simulink library "vmc"  (R2021b)
settings: Solver=VariableStepAuto  StartTime=0.0  StopTime=10.0  RelTol=1e-3
undefined symbols (not defined in the file): AVMC_ACCDeltaTqGradeGn_X_deg, AVMC_ACCDeltaTqIGain4OVRD_X_kph, AVMC_ACCDeltaTqIGain4OVRD_Y_mps2, AVMC_ACCDeltaTqIGain_X_kph, AVMC_ACCDeltaTqIGain_Y_mps2, AVMC_ACCDeltaTqPGain_X_kph, AVMC_ACCDeltaTqPGain_Y_kph, AVMC_ACCGradeofst_X_G, AVMC_ACCGradeofst_Y_pct, AVMC_ACCLoSpdTqLoLim4JP_X_kph, AVMC_ACCLoSpdTqLoLim4JP_Y_deg, AVMC_ACCLoSpdTqLowerLim_X_kph, AVMC_ACCLoSpdTqLowerLim_Y_deg, AVMC_ACCReqAccelGain_X_mps2, AVMC_ACCReqAccelGain_Y_enum, AVMC_ADSPosGFBDeltaTq_X_kph, AVMC_ADSPosGFBDeltaTq_Y_mps2, AVMC_AggressJerkPCT4AT_X_kph, AVMC_AggressJerkPCT_X_kph, AVMC_AggressLimitPCT4AT_X_kph, AVMC_AggressLimitPCT_X_kph, AVMC_DECGradeofst_X_G, AVMC_DECGradeofst_Y_pct, AVMC_DISCDeltaTqIGain_X_kph, AVMC_DISCDeltaTqIGain_Y_mps2, AVMC_DISCDeltaTqPGain_X_kph, AVMC_DISCDeltaTqPGain_Y_kph, AVMC_EPSForceSelect_X_enum, AVMC_EPSForceSelect_Y_enum, AVMC_EPSForceSelectD21_X_enum, AVMC_EPSForceSelectD21_Y_enum, AVMC_ESCRegenOut_X_kph, AVMC_ESCRegenOut_Y_Deg, AVMC_ESCRegenOutEnSpd_X_Deg, AVMC_EstPitchSlopeTs_X_kph, AVMC_GradeCompFlt_X_kph, AVMC_GyroYBandLo_X_Gps, AVMC_HoldResTq_X_kph, AVMC_ISOAccLimit_X_mps, AVMC_ISODecLimit_X_mps, AVMC_ISOJerk_X_mps, AVMC_LatESCRegenOut_X_kph, AVMC_LatESCRegenOut_Y_Deg, AVMC_LongAccDeadZone_X_kph, AVMC_LongAccFiltTsforP2_X_Gps, AVMC_MCPresBaseTq_X_bar, AVMC_MSAPedalOvrd_X_kph, AVMC_MSASpdBand_X_kph, AVMC_MSATqDownEndTq_X_kph, AVMC_MSATqDownTime_X_kph, AVMC_NegZCHoldTq_X_kph, AVMC_OPDDisSlideRate_X_Deg, AVMC_OVRD2ActSR2FCMCMD_X_mps2, AVMC_PedalTqRWhlRatio_X_Nm, AVMC_PedalTqRWhlRatio_Y_gps, AVMC_PedalTqRWhlSlipGain_X_rat, AVMC_PedalTqRWhlSlipGain_Y_kph, AVMC_PedalTqRWhSTRGGain_X_deg, AVMC_PedalTqRWhSTRGGain_Y_kph, AVMC_PosZCHoldTq_X_kph ... (+593)
libraries: hcu_lib x143, simulink x96, tqr x4, $bdroot x1, simulink_extras x1
(part 14 of 17)

== system vmc/VMC/VMC/Slide Rate  Calculation/Coordination ==
  VTQD_AfterAvailableTqDemFr_Nm : Inport
  VTQD_EquivAccPedalSWSta_flg : Inport  Port=2
  VINP_BrkPedalPos_pct : Inport  Port=3
  VVMC_PredictVehSpd_kph : Inport  Port=4
  VVMC_VehicleSpeed_kph : Inport  Port=5
  task_time_s : Inport  Port=6
  VINP_BrkSwSta_flg : Inport  Port=7
  VVMC_RawWhlSpdSlideRate_pct : Inport  Port=8
  VVMC_LFWhlSpdSlideRate_pct : Inport  Port=9
  VVMC_RFWhlSpdSlideRate_pct : Inport  Port=10
  VVMC_LRWhlSpdSlideRate_pct : Inport  Port=11
  VVMC_RRWhlSpdSlideRate_pct : Inport  Port=12
  VVMC_4WhlSpdSlideRate_pct : Inport  Port=13
  VVMC_LF4WhlSpdSlideRate_pct : Inport  Port=14
  VVMC_RF4WhlSpdSlideRate_pct : Inport  Port=15
  VVMC_LR4WhlSpdSlideRate_pct : Inport  Port=16
  VVMC_RR4WhlSpdSlideRate_pct : Inport  Port=17
  VVMC_AllWhlSkid_flg : Inport  Port=18
  VTQD_AfterAvailableTqDemRr_Nm : Inport  Port=19
  VVMC_AltWhlSlideRate_pct : Inport  Port=20
  VTQD_VehActSpd_kph : Inport  Port=21
  VTQD_RegenMode_enum : Inport  Port=22
  VVMC_EstSlope_Deg : Inport  Port=23
  AND : Logic  Inputs=4  AllPortsSameDT=off  OutDataTypeStr=boolean
  AND1 : Logic  AllPortsSameDT=off  OutDataTypeStr=boolean
  AND2 : Logic  AllPortsSameDT=off  OutDataTypeStr=boolean
  AND3 : Logic  Inputs=5  AllPortsSameDT=off  OutDataTypeStr=boolean
  Abs : Abs
  Abs1 : Abs
  Add : Sum  Inputs=+-
  Constant1 : Constant  Value=KVMC_WhlSlideEnDetTq_Nm
  Constant10 : Constant  Value=KVMC_WhlSlideEnDetTq_Nm
  Constant11 : Constant  Value=KVMC_AltWheelSlideRateSW_flg
  Constant{12..16} (5 alike) : Constant  Value=KVMC_CalWhleelSlideTs_c
  Constant17 : Constant  Value=KVMC_AltWheelSlideRateSW_flg
  Constant18 : Constant  Value=ZERO_FLOAT
  Constant19 : Constant  Value=KVMC_OPDDisSlideRateSpd_kph
  Constant2 : Constant  Value=KVMC_WhlSlideEnDetBrkPedal_pct
  Constant20 : Constant  Value=ENUM_REGENLEVEL_OPD
  Constant21 : Constant  Value=ZERO_FLOAT
  Constant{6..9,22} (5 alike) : Constant  Value=ONE_FLOAT
  Constant3 : Constant  Value=KVMC_4WhlSlideVehSpdDev_kph
  Constant4 : Constant  Value=KVMC_WhlSlideEnDetVehSpd_kph
  Constant5 : Constant  Value=KVMC_4WhleelSlideDetTime_s
  DelayEnable : hcu_lib/Basic_Blocks/DelayEnable
  Equal : RelationalOperator  Operator===  OutDataTypeStr=boolean  RndMeth=Simplest
  FirstOrderFilter{,1..4} (5 alike) : hcu_lib/Basic_Blocks/FirstOrderFilter
  MVMC_OPDDisSlideRate_Y_pct : Lookup_n-D  NumberOfTableDimensions=1  BreakpointsForDimension1=AVMC_OPDDisSlideRate_X_Deg  Table=MVMC_OPDDisSlideRate_Y_pct  InternalRulePriority=Speed  RndMeth=Simplest  InputSameDT=on
  NOT{,1..3} (4 alike) : Logic  Operator=NOT  AllPortsSameDT=off  OutDataTypeStr=boolean
  OR : Logic  Operator=OR  Inputs=3  AllPortsSameDT=off  OutDataTypeStr=boolean
  Relational Operator{,1,3..4,7} (5 alike) : RelationalOperator  OutDataTypeStr=boolean  RndMeth=Simplest
  Relational Operator2 : RelationalOperator  Operator=<  OutDataTypeStr=boolean  RndMeth=Simplest
  Relational Operator5 : RelationalOperator  Operator=<=  OutDataTypeStr=boolean  RndMeth=Simplest
  Relational Operator6 : RelationalOperator  Operator=<  OutDataTypeStr=boolean  RndMeth=Simplest
  Relay : Relay  OnSwitchValue=KTQD_OPDHoldGradeUp_Deg  OffSwitchValue=KTQD_OPDHoldGradeDown_Deg  OutDataTypeStr=boolean
  Switch{,1..11} (12 alike) : Switch  Criteria=u2 > Threshold
  VVMC_ActMaxSlideRate_pct : Outport
  VVMC_ActLFSlideRate_pct : Outport  Port=2
  VVMC_ActRFSlideRate_pct : Outport  Port=3
  VVMC_ActLRSlideRate_pct : Outport  Port=4
  VVMC_ActRRSlideRate_pct : Outport  Port=5
  wires:
  [VVMC_SlideRateEnCal_flg] -> Switch9/2
  [VVMC_SlideRateEnCal_flg] -> Switch7/2
  [VVMC_SlideRateEnCal_flg] -> Switch5/2
  [VVMC_SlideRateEnCal_flg] -> Switch3/2
  [VVMC_SlideRateEnCal_flg] -> Switch1/2
  [VVMC_EstSlope_Deg] -> Relay/1
  Relay/1 -> NOT3/1
  NOT3/1 -> AND3/5
  Relational Operator7/1 -> AND3/4
  [VTQD_VehActSpd_kph] -> Relational Operator7/1
  Constant22/1 -> Relational Operator7/2
  Constant21/1 -> Switch11/1
  [VVMC_OPDDisSlideRate_flg] -> Switch11/2
  Switch11/1 -> [VVMC_ActMaxSlideRate_pct]  "VVMC_ActMaxSlideRate_pct"
  FirstOrderFilter/1 -> Switch11/3, [VVMC_IntMaxSlideRate_pct]  "VVMC_IntMaxSlideRate_pct"
  Abs1/1 -> Relational Operator6/1
  [VVMC_IntMaxSlideRate_pct] -> Abs1/1
  AND3/1 -> [VVMC_OPDDisSlideRate_flg]  "VVMC_OPDDisSlideRate_flg"
  Relational Operator6/1 -> AND3/3
  Equal/1 -> AND3/2
  Relational Operator5/1 -> AND3/1
  MVMC_OPDDisSlideRate_Y_pct/1 -> Relational Operator6/2  "VVMC_OPDDisSlideRate_pct"
  [VVMC_EstSlope_Deg] -> MVMC_OPDDisSlideRate_Y_pct/1
  Constant20/1 -> Equal/2
  [VTQD_RegenMode_enum] -> Equal/1
  Constant19/1 -> Relational Operator5/2
  [VTQD_VehActSpd_kph] -> Relational Operator5/1
  VTQD_VehActSpd_kph/1 -> [VTQD_VehActSpd_kph]
  VTQD_RegenMode_enum/1 -> [VTQD_RegenMode_enum]
  VVMC_EstSlope_Deg/1 -> [VVMC_EstSlope_Deg]
  AND2/1 -> Switch/2
  NOT2/1 -> AND2/2
  Constant17/1 -> NOT2/1
  [task_time_s] -> FirstOrderFilter4/2
  Constant16/1 -> FirstOrderFilter4/3
  [task_time_s] -> FirstOrderFilter3/2
  Constant15/1 -> FirstOrderFilter3/3
  Constant14/1 -> FirstOrderFilter2/3
  [task_time_s] -> FirstOrderFilter2/2
  Constant13/1 -> FirstOrderFilter1/3
  [task_time_s] -> FirstOrderFilter1/2
  [task_time_s] -> FirstOrderFilter/2
  Constant12/1 -> FirstOrderFilter/3
  FirstOrderFilter4/1 -> [VVMC_ActRRSlideRate_pct]  "VVMC_ActRRSlideRate_pct"
  Switch9/1 -> FirstOrderFilter4/1
  FirstOrderFilter3/1 -> [VVMC_ActLRSlideRate_pct]  "VVMC_ActLRSlideRate_pct"
  Switch7/1 -> FirstOrderFilter3/1
  FirstOrderFilter2/1 -> [VVMC_ActRFSlideRate_pct]  "VVMC_ActRFSlideRate_pct"
  Switch5/1 -> FirstOrderFilter2/1
  Switch3/1 -> FirstOrderFilter1/1
  FirstOrderFilter1/1 -> [VVMC_ActLFSlideRate_pct]  "VVMC_ActLFSlideRate_pct"
  Switch1/1 -> FirstOrderFilter/1
  Constant11/1 -> Switch10/2
  [VVMC_AltWhlSlideRate_pct] -> Switch10/1
  Switch10/1 -> Switch/3
  [VVMC_RawWhlSpdSlideRate_pct] -> Switch10/3
  VVMC_AltWhlSlideRate_pct/1 -> [VVMC_AltWhlSlideRate_pct]
  VTQD_AfterAvailableTqDemRr_Nm/1 -> [VTQD_AfterAvailableTqDemRr_Nm]
  [VTQD_AfterAvailableTqDemFr_Nm] -> Relational Operator1/1
  Relational Operator4/1 -> OR/1
  Relational Operator1/1 -> OR/2
  NOT/1 -> OR/3
  [VTQD_AfterAvailableTqDemRr_Nm] -> Relational Operator4/1
  Constant10/1 -> Relational Operator4/2
  [VVMC_AllWhlSkid_flg] -> AND1/1
  AND1/1 -> [VVMC_4WheelSlide_flg]  "VVMC_4WheelSlide_flg"
  DelayEnable/1 -> AND1/2  "VVMC_VehSpdPredSkid_flg"
  VVMC_AllWhlSkid_flg/1 -> [VVMC_AllWhlSkid_flg]
  [task_time_s] -> DelayEnable/3
  Constant2/1 -> Relational Operator2/2
  Constant3/1 -> Relational Operator/2
  AND/1 -> [VVMC_SlideRateEnCal_flg]  "VVMC_SlideRateEnCal_flg"
  Relational Operator2/1 -> AND/2
  [VVMC_VehicleSpeed_kph] -> Relational Operator3/1
  [VINP_BrkSwSta_flg] -> NOT1/1
  [VVMC_PredictVehSpd_kph] -> Add/1
  Constant1/1 -> Relational Operator1/2
  [VVMC_LFWhlSpdSlideRate_pct] -> Switch2/3
  Relational Operator3/1 -> AND/4
  [VVMC_RR4WhlSpdSlideRate_pct] -> Switch8/1
  [VVMC_4WheelSlide_flg] -> Switch8/2
  Relational Operator/1 -> DelayEnable/1
  [VVMC_4WheelSlide_flg] -> Switch2/2
  Add/1 -> Abs/1
  [VVMC_4WheelSlide_flg] -> Switch4/2
  [VVMC_RF4WhlSpdSlideRate_pct] -> Switch4/1
  Switch2/1 -> Switch3/1
  Constant6/1 -> Switch3/3
  Constant18/1 -> Switch1/3
  [VVMC_RFWhlSpdSlideRate_pct] -> Switch4/3
  NOT1/1 -> AND/3
  Switch6/1 -> Switch7/1
  [VINP_BrkPedalPos_pct] -> Relational Operator2/1
  Constant5/1 -> DelayEnable/2
  Constant9/1 -> Switch9/3
  Switch4/1 -> Switch5/1
  Constant7/1 -> Switch5/3
  Switch/1 -> Switch1/1
  [VVMC_LRWhlSpdSlideRate_pct] -> Switch6/3
  Switch8/1 -> Switch9/1
  Abs/1 -> Relational Operator/1
  [VVMC_LF4WhlSpdSlideRate_pct] -> Switch2/1
  Constant8/1 -> Switch7/3
  [VTQD_EquivAccPedalSWSta_flg] -> NOT/1
  [VVMC_LR4WhlSpdSlideRate_pct] -> Switch6/1
  [VVMC_4WheelSlide_flg] -> Switch6/2
  [VVMC_4WhlSpdSlideRate_pct] -> Switch/1
  [VVMC_4WheelSlide_flg] -> AND2/1
  Constant4/1 -> Relational Operator3/2
  [VVMC_RRWhlSpdSlideRate_pct] -> Switch8/3
  OR/1 -> AND/1
  [VVMC_VehicleSpeed_kph] -> Add/2
  [VVMC_ActRRSlideRate_pct] -> VVMC_ActRRSlideRate_pct/1
  [VVMC_ActLRSlideRate_pct] -> VVMC_ActLRSlideRate_pct/1
  [VVMC_ActMaxSlideRate_pct] -> VVMC_ActMaxSlideRate_pct/1
  [VVMC_ActLFSlideRate_pct] -> VVMC_ActLFSlideRate_pct/1
  [VVMC_ActRFSlideRate_pct] -> VVMC_ActRFSlideRate_pct/1
  VVMC_PredictVehSpd_kph/1 -> [VVMC_PredictVehSpd_kph]
  VTQD_AfterAvailableTqDemFr_Nm/1 -> [VTQD_AfterAvailableTqDemFr_Nm]
  VTQD_EquivAccPedalSWSta_flg/1 -> [VTQD_EquivAccPedalSWSta_flg]
  VINP_BrkPedalPos_pct/1 -> [VINP_BrkPedalPos_pct]
  VVMC_VehicleSpeed_kph/1 -> [VVMC_VehicleSpeed_kph]
  VINP_BrkSwSta_flg/1 -> [VINP_BrkSwSta_flg]
  task_time_s/1 -> [task_time_s]
  VVMC_RawWhlSpdSlideRate_pct/1 -> [VVMC_RawWhlSpdSlideRate_pct]
  VVMC_RFWhlSpdSlideRate_pct/1 -> [VVMC_RFWhlSpdSlideRate_pct]
  VVMC_LFWhlSpdSlideRate_pct/1 -> [VVMC_LFWhlSpdSlideRate_pct]
  VVMC_RRWhlSpdSlideRate_pct/1 -> [VVMC_RRWhlSpdSlideRate_pct]
  VVMC_LRWhlSpdSlideRate_pct/1 -> [VVMC_LRWhlSpdSlideRate_pct]
  VVMC_4WhlSpdSlideRate_pct/1 -> [VVMC_4WhlSpdSlideRate_pct]
  VVMC_LF4WhlSpdSlideRate_pct/1 -> [VVMC_LF4WhlSpdSlideRate_pct]
  VVMC_RF4WhlSpdSlideRate_pct/1 -> [VVMC_RF4WhlSpdSlideRate_pct]
  VVMC_LR4WhlSpdSlideRate_pct/1 -> [VVMC_LR4WhlSpdSlideRate_pct]
  VVMC_RR4WhlSpdSlideRate_pct/1 -> [VVMC_RR4WhlSpdSlideRate_pct]

== system vmc/VMC/VMC/Slide Rate  Calculation/Partial Wheel Calculation ==
  VINP_LFRawWhlSpeed_kph : Inport
  VINP_RFRawWhlSpeed_kph : Inport  Port=2
  VINP_LRRawWhlSpeed_kph : Inport  Port=3
  VINP_RRRawWhlSpeed_kph : Inport  Port=4
  VTQD_AfterAvailableTqDemFr_Nm : Inport  Port=5
  VTQD_AfterAvailableTqDemRr_Nm : Inport  Port=6
  Add{,1..4} (5 alike) : Sum  Inputs=+-
  Add5 : Sum
  Constant{,3,5,8,10,13,15,18,20,23} (10 alike) : Constant  Value=KVMC_RawWhlSpeedDeadZone_kph
  Constant{1,6,11,16,21,26} (6 alike) : Constant  Value=ONE_FLOAT
  Constant{2,7,12,17,22} (5 alike) : Constant  Value=ONE_PERCENT
  Constant{4,9,14,19,24..25} (6 alike) : Constant  Value=ZERO_FLOAT
  Constant27 : Constant  Value=MINUSONE_FLOAT
  Divide{,1..4} (5 alike) : Product  Inputs=*//
  Max : MinMax  Function=max  Inputs=4
  Max1 : MinMax  Inputs=4
  Product : Product
  Relational Operator{,1..10} (11 alike) : RelationalOperator  Operator=<=  OutDataTypeStr=boolean  RndMeth=Simplest
  Switch{,1..10} (11 alike) : Switch  Criteria=u2 > Threshold
  VVMC_RawWhlSpdSlideRate_pct : Outport
  VVMC_LFWhlSpdSlideRate_pct : Outport  Port=2
  VVMC_RFWhlSpdSlideRate_pct : Outport  Port=3
  VVMC_LRWhlSpdSlideRate_pct : Outport  Port=4
  VVMC_RRWhlSpdSlideRate_pct : Outport  Port=5
  wires:
  Switch10/1 -> Product/1
  Switch1/1 -> Product/2
  Constant25/1 -> Relational Operator10/2
  Constant26/1 -> Switch10/3
  Add5/1 -> Relational Operator10/1
  [VTQD_AfterAvailableTqDemFr_Nm] -> Add5/1
  [VTQD_AfterAvailableTqDemRr_Nm] -> Add5/2
  Constant27/1 -> Switch10/1
  Relational Operator10/1 -> Switch10/2
  VTQD_AfterAvailableTqDemRr_Nm/1 -> [VTQD_AfterAvailableTqDemRr_Nm]
  VTQD_AfterAvailableTqDemFr_Nm/1 -> [VTQD_AfterAvailableTqDemFr_Nm]
  [VVMC_MinRawWhlSpeed_kph] -> Relational Operator8/1
  [VVMC_MinRawWhlSpeed_kph] -> Relational Operator/1
  Constant5/1 -> Relational Operator2/2
  Divide/1 -> Switch1/3  "VVMC_RawCalWhlSpdSlideRate_pct"
  Relational Operator8/1 -> Switch8/2
  Relational Operator5/1 -> Switch5/2
  [VVMC_MinRawWhlSpeed_kph] -> Add/2
  Switch5/1 -> [VVMC_RFWhlSpdSlideRate_pct]  "VVMC_RFWhlSpdSlideRate_pct"
  Constant4/1 -> Switch1/1
  Switch8/1 -> Divide4/3
  Switch/1 -> Divide/3
  Relational Operator9/1 -> Switch9/2
  Constant20/1 -> Relational Operator8/2
  Constant1/1 -> Switch/1
  [VVMC_MinRawWhlSpeed_kph] -> Add4/2
  [VVMC_MinRawWhlSpeed_kph] -> Add1/2
  [VVMC_MaxRawWhlSpeed_kph] -> Relational Operator1/1
  Relational Operator/1 -> Switch/2
  Divide4/1 -> Switch9/3  "VVMC_RRCalWhlSpdSlideRate_pct"
  Constant/1 -> Relational Operator/2
  Constant10/1 -> Relational Operator4/2
  [VVMC_MinRawWhlSpeed_kph] -> Relational Operator2/1
  [VINP_RFRawWhlSpeed_kph] -> Relational Operator5/1
  [VVMC_MinRawWhlSpeed_kph] -> Switch8/3
  Switch9/1 -> [VVMC_RRWhlSpdSlideRate_pct]  "VVMC_RRWhlSpdSlideRate_pct"
  Relational Operator2/1 -> Switch2/2
  [VINP_RRRawWhlSpeed_kph] -> Add4/1
  Constant3/1 -> Relational Operator1/2
  Add1/1 -> Divide1/1
  Constant23/1 -> Relational Operator9/2
  Constant13/1 -> Relational Operator5/2
  [VINP_LFRawWhlSpeed_kph] -> Add1/1
  [VVMC_MinRawWhlSpeed_kph] -> Switch2/3
  [VINP_LFRawWhlSpeed_kph] -> Max1/1
  Constant19/1 -> Switch7/1
  Max/1 -> [VVMC_MaxRawWhlSpeed_kph]  "VVMC_MaxRawWhlSpeed_kph"
  Constant6/1 -> Switch2/1
  [VVMC_MinRawWhlSpeed_kph] -> Switch4/3
  [VINP_RRRawWhlSpeed_kph] -> Max1/4
  Divide2/1 -> Switch5/3  "VVMC_RFCalWhlSpdSlideRate_pct"
  Switch2/1 -> Divide1/3
  Relational Operator1/1 -> Switch1/2
  [VVMC_MinRawWhlSpeed_kph] -> Relational Operator4/1
  [VINP_LRRawWhlSpeed_kph] -> Max/3
  [VVMC_MaxRawWhlSpeed_kph] -> Add/1
  [VVMC_MinRawWhlSpeed_kph] -> Add2/2
  Add2/1 -> Divide2/1
  Relational Operator4/1 -> Switch4/2
  [VINP_RFRawWhlSpeed_kph] -> Max/2
  [VINP_RFRawWhlSpeed_kph] -> Add2/1
  Constant11/1 -> Switch4/1
  Divide3/1 -> Switch7/3  "VVMC_LRCalWhlSpdSlideRate_pct"
  Constant12/1 -> Divide2/2
  Switch4/1 -> Divide2/3
  Constant22/1 -> Divide4/2
  Constant21/1 -> Switch8/1
  Constant9/1 -> Switch3/1
  Constant14/1 -> Switch5/1
  [VINP_RRRawWhlSpeed_kph] -> Max/4
  [VINP_LFRawWhlSpeed_kph] -> Max/1
  Constant24/1 -> Switch9/1
  Add4/1 -> Divide4/1
  [VVMC_MinRawWhlSpeed_kph] -> Switch/3
  [VINP_RRRawWhlSpeed_kph] -> Relational Operator9/1
  Relational Operator3/1 -> Switch3/2
  Constant2/1 -> Divide/2
  Product/1 -> [VVMC_RawWhlSpdSlideRate_pct]  "VVMC_RawWhlSpdSlideRate_pct"
  Constant7/1 -> Divide1/2
  Constant8/1 -> Relational Operator3/2
  Switch3/1 -> [VVMC_LFWhlSpdSlideRate_pct]  "VVMC_LFWhlSpdSlideRate_pct"
  [VINP_LFRawWhlSpeed_kph] -> Relational Operator3/1
  Divide1/1 -> Switch3/3  "VVMC_LFCalWhlSpdSlideRate_pct"
  Add/1 -> Divide/1
  Max1/1 -> [VVMC_MinRawWhlSpeed_kph]  "VVMC_MinRawWhlSpeed_kph"
  [VINP_LRRawWhlSpeed_kph] -> Max1/3
  [VINP_RFRawWhlSpeed_kph] -> Max1/2
  [VVMC_MinRawWhlSpeed_kph] -> Add3/2
  Add3/1 -> Divide3/1
  [VINP_LRRawWhlSpeed_kph] -> Add3/1
  [VVMC_MinRawWhlSpeed_kph] -> Relational Operator6/1
  [VVMC_MinRawWhlSpeed_kph] -> Switch6/3
  Constant18/1 -> Relational Operator7/2
  [VINP_LRRawWhlSpeed_kph] -> Relational Operator7/1
  Relational Operator7/1 -> Switch7/2
  Switch7/1 -> [VVMC_LRWhlSpdSlideRate_pct]  "VVMC_LRWhlSpdSlideRate_pct"
  Switch6/1 -> Divide3/3
  Constant17/1 -> Divide3/2
  Constant16/1 -> Switch6/1
  Relational Operator6/1 -> Switch6/2
  Constant15/1 -> Relational Operator6/2
  VINP_LFRawWhlSpeed_kph/1 -> [VINP_LFRawWhlSpeed_kph]
  VINP_RFRawWhlSpeed_kph/1 -> [VINP_RFRawWhlSpeed_kph]
  VINP_LRRawWhlSpeed_kph/1 -> [VINP_LRRawWhlSpeed_kph]
  VINP_RRRawWhlSpeed_kph/1 -> [VINP_RRRawWhlSpeed_kph]
  [VVMC_RawWhlSpdSlideRate_pct] -> VVMC_RawWhlSpdSlideRate_pct/1
  [VVMC_RFWhlSpdSlideRate_pct] -> VVMC_RFWhlSpdSlideRate_pct/1
  [VVMC_LFWhlSpdSlideRate_pct] -> VVMC_LFWhlSpdSlideRate_pct/1
  [VVMC_LRWhlSpdSlideRate_pct] -> VVMC_LRWhlSpdSlideRate_pct/1
  [VVMC_RRWhlSpdSlideRate_pct] -> VVMC_RRWhlSpdSlideRate_pct/1

== system vmc/VMC/VMC/SpeedArbitration/Feature Arbitration ==
  VVMC_FeatStaConfirm_enum : Inport
  VDSC_DISCTargetSpd_kph : Inport  Port=2
  VVMC_FeatSetSpdForCalcu_kph : Inport  Port=3
  VDSC_PreACC_flg : Inport  Port=4
  Constant1 : Constant  Value=ENUM_FEATSTACFM_AEB
  Constant10 : Constant  Value=ENUM_FEATARBITRSTA_AEB
  Constant11 : Constant  Value=ENUM_FEATARBITRSTA_ACC
  Constant12 : Constant  Value=ENUM_FEATARBITRSTA_CC
  Constant13 : Constant  Value=ENUM_FEATARBITRSTA_DISC
  Constant14 : Constant  Value=ENUM_FEATARBITRSTA_MSA
  Constant15 : Constant  Value=ZERO_FLOAT
  Constant18 : Constant  Value=ENUM_FEATARBITRSTA_ACCDISC
  Constant2 : Constant  Value=ENUM_FEATSTACFM_ACC
  Constant3 : Constant  Value=ENUM_FEATSTACFM_CC
  Constant4 : Constant  Value=ENUM_FEATSTACFM_DISC
  Constant5 : Constant  Value=ENUM_FEATSTACFM_MSA
  Constant6 : Constant  Value=ENUM_FEATSTACFM_ACCDISC
  Constant7 : Constant  Value=ENUM_FEATSTACFM_CCDISC
  Constant8 : Constant  Value=ENUM_FEATSTACFM_DISCMSA
  Constant9 : Constant  Value=ENUM_FEATARBITRSTA_INACTIVE
  Feature Arbitration : Stateflow chart  TreatAsAtomicUnit=on
  VVMC_FeatArbitrSta_enum : Outport
  VVMC_FeatReqSpd_kph : Outport  Port=2
  wires:
  VDSC_PreACC_flg/1 -> [VDSC_PreACC_flg]
  [VDSC_PreACC_flg] -> Feature Arbitration/20(VDSC_PreACC_flg)
  VVMC_FeatStaConfirm_enum/1 -> [VVMC_FeatStaConfirm_enum]
  VDSC_DISCTargetSpd_kph/1 -> [VDSC_DISCTargetSpd_kph]
  VVMC_FeatSetSpdForCalcu_kph/1 -> [VVMC_FeatSetSpdForCalcu_kph]
  [VVMC_FeatStaConfirm_enum] -> Feature Arbitration/1(VVMC_FeatStaConfirm_enum)
  [VDSC_DISCTargetSpd_kph] -> Feature Arbitration/2(VDSC_DISCTargetSpd_kph)
  [VVMC_FeatSetSpdForCalcu_kph] -> Feature Arbitration/3(VVMC_FeatSetSpdForCalcu_kph)
  Feature Arbitration/1(VVMC_FeatArbitrSta_enum) -> [VVMC_FeatArbitrSta_enum]
  Feature Arbitration/2(VVMC_FeatReqSpd_kph) -> [VVMC_FeatReqSpd_kph]
  [VVMC_FeatArbitrSta_enum] -> VVMC_FeatArbitrSta_enum/1
  [VVMC_FeatReqSpd_kph] -> VVMC_FeatReqSpd_kph/1
  Constant1/1 -> Feature Arbitration/4(ENUM_FEATSTACFM_AEB)
  Constant2/1 -> Feature Arbitration/5(ENUM_FEATSTACFM_ACC)
  Constant3/1 -> Feature Arbitration/6(ENUM_FEATSTACFM_CC)
  Constant4/1 -> Feature Arbitration/7(ENUM_FEATSTACFM_DISC)
  Constant5/1 -> Feature Arbitration/8(ENUM_FEATSTACFM_MSA)
  Constant6/1 -> Feature Arbitration/9(ENUM_FEATSTACFM_ACCDISC)
  Constant7/1 -> Feature Arbitration/10(ENUM_FEATSTACFM_CCDISC)
  Constant8/1 -> Feature Arbitration/11(ENUM_FEATSTACFM_DISCMSA)
  Constant9/1 -> Feature Arbitration/12(ENUM_FEATARBITRSTA_INACTIVE)
  Constant10/1 -> Feature Arbitration/13(ENUM_FEATARBITRSTA_AEB)
  Constant11/1 -> Feature Arbitration/14(ENUM_FEATARBITRSTA_ACC)
  Constant12/1 -> Feature Arbitration/15(ENUM_FEATARBITRSTA_CC)
  Constant13/1 -> Feature Arbitration/16(ENUM_FEATARBITRSTA_DISC)
  Constant14/1 -> Feature Arbitration/18(ENUM_FEATARBITRSTA_MSA)
  Constant15/1 -> Feature Arbitration/19(ZERO_FLOAT)
  Constant18/1 -> Feature Arbitration/17(ENUM_FEATARBITRSTA_ACCDISC)

== system vmc/VMC/VMC/SpeedArbitration/Feature Status Confirm ==
  VVMC_VMCCCCtrlAvail_flg : Inport
  VVMC_VMCMSACtrlAvail_flg : Inport  Port=2
  VVMC_VMCAEBCtrlAvail_flg : Inport  Port=3
  VVMC_VMCACCCtrlAvail_flg : Inport  Port=4
  VINP_ADASAEBSta_enum : Inport  Port=5
  VDSC_DISCSta_enum : Inport  Port=6
  VINP_ADASACCSta_enum : Inport  Port=7
  VVMC_CCCtrlSta_enum : Inport  Port=8
  VVMC_MSACtrlSta_enum : Inport  Port=9
  VINP_ADASAEBReq_enum : Inport  Port=10
  VDSC_PreACC_flg : Inport  Port=11
  Constant : Constant  Value=ENUM_FEATSTACFM_INACTIVE
  Constant1 : Constant  Value=ENUM_FEATSTACFM_AEB
  Constant10 : Constant  Value=ENUM_VMCAEBCTRLAVAIL_AVAILABLE
  Constant11 : Constant  Value=ENUM_CCCRLSTA_ACTIVE
  Constant12 : Constant  Value=ENUM_ADASMSASTA_ACTIVE
  Constant13 : Constant  Value=ENUM_DISCSTA_ACTIVE
  Constant14 : Constant  Value=ENUM_ADASAEBSTA_ACTIVE
  Constant15 : Constant  Value=ENUM_VMCACCCTRLAVAIL_AVAILABLE
  Constant16 : Constant  Value=ENUM_VMCMSACTRLAVAIL_AVAILABLE
  Constant17 : Constant  Value=ENUM_VMCCCCTRLAVAIL_AVAILABLE
  Constant18 : Constant  Value=ENUM_ADASACCSTA_SHUTOFF
  Constant19 : Constant  Value=ENUM_ADASACCSTA_OVERRIDE
  Constant2 : Constant  Value=ENUM_FEATSTACFM_ACC
  Constant20 : Constant  Value=ENUM_ADASAEBREQ_NOREQUEST
  Constant21 : Constant  Value=ENUM_CCCRLSTA_OVERRIDE
  Constant22 : Constant  Value=ENUM_ADASMSASTA_UNLIMIT
  Constant3 : Constant  Value=ENUM_FEATSTACFM_CC
  Constant4 : Constant  Value=ENUM_FEATSTACFM_DISC
  Constant5 : Constant  Value=ENUM_FEATSTACFM_MSA
  Constant6 : Constant  Value=ENUM_FEATSTACFM_ACCDISC
  Constant7 : Constant  Value=ENUM_FEATSTACFM_CCDISC
  Constant8 : Constant  Value=ENUM_FEATSTACFM_DISCMSA
  Constant9 : Constant  Value=ENUM_ADASACCSTA_ACTIVE
  Feature Status Confirm : Stateflow chart  TreatAsAtomicUnit=on
  VVMC_FeatStaConfirm_enum : Outport
  wires:
  VDSC_PreACC_flg/1 -> [VDSC_PreACC_flg]
  [VDSC_PreACC_flg] -> Feature Status Confirm/34(VDSC_PreACC_flg)
  Constant21/1 -> Feature Status Confirm/32(ENUM_CCCRLSTA_OVERRIDE)
  Constant22/1 -> Feature Status Confirm/33(ENUM_MSACRLSTA_OVERRIDE)
  [VVMC_MSACtrlSta_enum] -> Feature Status Confirm/13(VVMC_MSACtrlSta_enum)
  [VDSC_DISCSta_enum] -> Feature Status Confirm/10(VDSC_DISCSta_enum)
  [VINP_ADASACCSta_enum] -> Feature Status Confirm/11(VINP_ADASACCSta_enum)
  [VINP_ADASAEBSta_enum] -> Feature Status Confirm/9(VINP_ADASAEBSta_enum)
  [VVMC_CCCtrlSta_enum] -> Feature Status Confirm/12(VVMC_CCCtrlSta_enum)
  VINP_ADASAEBSta_enum/1 -> [VINP_ADASAEBSta_enum]
  VDSC_DISCSta_enum/1 -> [VDSC_DISCSta_enum]
  VINP_ADASACCSta_enum/1 -> [VINP_ADASACCSta_enum]
  VVMC_CCCtrlSta_enum/1 -> [VVMC_CCCtrlSta_enum]
  VVMC_MSACtrlSta_enum/1 -> [VVMC_MSACtrlSta_enum]
  Feature Status Confirm/1(VVMC_FeatStaConfirm_enum) -> [VVMC_FeatStaConfirm_enum]
  [VVMC_FeatStaConfirm_enum] -> VVMC_FeatStaConfirm_enum/1
  Constant/1 -> Feature Status Confirm/14(ENUM_FEATSTACFM_INACTIVE)
  Constant1/1 -> Feature Status Confirm/15(ENUM_FEATSTACFM_AEB)
  Constant2/1 -> Feature Status Confirm/16(ENUM_FEATSTACFM_ACC)
  Constant3/1 -> Feature Status Confirm/17(ENUM_FEATSTACFM_CC)
  Constant4/1 -> Feature Status Confirm/18(ENUM_FEATSTACFM_DISC)
  Constant5/1 -> Feature Status Confirm/19(ENUM_FEATSTACFM_MSA)
  Constant6/1 -> Feature Status Confirm/20(ENUM_FEATSTACFM_ACCDISC)
  Constant7/1 -> Feature Status Confirm/21(ENUM_FEATSTACFM_CCDISC)
  Constant8/1 -> Feature Status Confirm/22(ENUM_FEATSTACFM_DISCMSA)
  Constant9/1 -> Feature Status Confirm/24(ENUM_ADASACCSTA_ACTIVE)
  Constant11/1 -> Feature Status Confirm/26(ENUM_CCCRLSTA_ACTIVE)
  Constant12/1 -> Feature Status Confirm/27(ENUM_MSACRLSTA_ACTIVE)
  Constant13/1 -> Feature Status Confirm/28(ENUM_DISCSTA_ACTIVE)
  Constant14/1 -> Feature Status Confirm/23(ENUM_ADASAEBSTA_ACTIVE)
  VVMC_VMCACCCtrlAvail_flg/1 -> [VVMC_VMCACCCtrlAvail_flg]
  VVMC_VMCAEBCtrlAvail_flg/1 -> [VVMC_VMCAEBCtrlAvail_flg]
  Constant15/1 -> Feature Status Confirm/8(ENUM_VMCACCCTRLAVAIL_AVAILABLE)
  [VVMC_VMCACCCtrlAvail_flg] -> Feature Status Confirm/7(VVMC_VMCACCCtrlAvail_flg)
  Constant10/1 -> Feature Status Confirm/6(ENUM_VMCAEBCTRLAVAIL_AVAILABLE)
  [VVMC_VMCAEBCtrlAvail_flg] -> Feature Status Confirm/5(VVMC_VMCAEBCtrlAvail_flg)
  VVMC_VMCCCCtrlAvail_flg/1 -> [VVMC_VMCCCCtrlAvail_flg]
  VVMC_VMCMSACtrlAvail_flg/1 -> [VVMC_VMCMSACtrlAvail_flg]
  Constant16/1 -> Feature Status Confirm/4(ENUM_VMCMSACTRLAVAIL_AVAILABLE)
  [VVMC_VMCMSACtrlAvail_flg] -> Feature Status Confirm/3(VVMC_VMCMSACtrlAvail_flg)
  Constant17/1 -> Feature Status Confirm/2(ENUM_VMCCCCTRLAVAIL_AVAILABLE)
  [VVMC_VMCCCCtrlAvail_flg] -> Feature Status Confirm/1(VVMC_VMCCCCtrlAvail_flg)
  Constant18/1 -> Feature Status Confirm/25(ENUM_ADASACCSTA_SHUTOFF)
  Constant19/1 -> Feature Status Confirm/29(ENUM_ADASACCSTA_OVERRIDE)
  VINP_ADASAEBReq_enum/1 -> [VINP_ADASAEBReq_enum]
  [VINP_ADASAEBReq_enum] -> Feature Status Confirm/30(VINP_ADASAEBReq_enum)
  Constant20/1 -> Feature Status Confirm/31(ENUM_ADASAEBREQ_NOREQUEST)

== system vmc/VMC/VMC/SpeedArbitration/Response Gain ==
  VDSC_DISCTurn_flg : Inport
  VVMC_FeatArbitrSta_enum : Inport  Port=2
  VVMC_FeatReqSpd_kph : Inport  Port=3
  VVMC_MeterIndSpeedForCalcu_kph : Inport  Port=4
  VVMC_VehicleSpeed_kph : Inport  Port=5
  VDSC_AutoTurnMode_flg : Inport  Port=6
  VDSC_DISCTargetSpd_kph : Inport  Port=7
  Abs : Abs
  Add : Sum  Inputs=-+
  Add4 : Sum
  Constant1 : Constant  Value=KVMC_Veh2MeterSpdFactor_enum
  Constant13 : Constant  Value=ENUM_FEATARBITRSTA_DISC
  Constant{15,29,31,33,35} (5 alike) : Constant  Value=ZERO_FLOAT
  Constant16 : Constant  Value=ENUM_DISCTURN_ACTIVE
  Constant18 : Constant  Value=ENUM_FEATARBITRSTA_ACCDISC
  Constant2 : Constant  Value=ENUM_FEATARBITRSTA_CC
  Constant23 : Constant  Value=KVMC_Veh2MeterSpdOffset_enum
  Constant28 : Constant  Value=KVMC_Veh2MeterSpdLoFactor_enum
  Constant3 : Constant  Value=ENUM_FEATARBITRSTA_MSA
  Constant{30,32,34,36} (4 alike) : Constant  Value=HUNDRED
  Constant4 : Constant  Value=TRUE
  Constant5 : Constant  Value=KVMC_MSAResponseAGSV_flg
  Divide5 : Product  Inputs=**
  Divide8 : Product  Inputs=**
  MVMC_AggressJerkPCT4AT_pct : Lookup_n-D  NumberOfTableDimensions=1  BreakpointsForDimension1=AVMC_AggressJerkPCT4AT_X_kph  Table=MVMC_AggressJerkPCT4AT_Y_pct  InternalRulePriority=Speed  RndMeth=Simplest  InputSameDT=on
  MVMC_AggressJerkPCT_pct : Lookup_n-D  NumberOfTableDimensions=1  BreakpointsForDimension1=AVMC_AggressJerkPCT_X_kph  Table=MVMC_AggressJerkPCT_Y_pct  InternalRulePriority=Speed  RndMeth=Simplest  InputSameDT=on
  MVMC_AggressJerkPCT_pct1 : Lookup_n-D  NumberOfTableDimensions=1  BreakpointsForDimension1=AVMC_AggressJerkPCT_X_kph  Table=MVMC_AggressJerkPCT_Y_pct  InternalRulePriority=Speed  RndMeth=Simplest  InputSameDT=on
  MVMC_AggressLimitPCT4AT_pct : Lookup_n-D  NumberOfTableDimensions=1  BreakpointsForDimension1=AVMC_AggressLimitPCT4AT_X_kph  Table=MVMC_AggressLimitPCT4AT_Y_pct  InternalRulePriority=Speed  RndMeth=Simplest  InputSameDT=on
  MVMC_AggressLimitPCT_pct : Lookup_n-D  NumberOfTableDimensions=1  BreakpointsForDimension1=AVMC_AggressLimitPCT_X_kph  Table=MVMC_AggressLimitPCT_Y_pct  InternalRulePriority=Speed  RndMeth=Simplest  InputSameDT=on
  MVMC_AggressLimitPCT_pct1 : Lookup_n-D  NumberOfTableDimensions=1  BreakpointsForDimension1=AVMC_AggressLimitPCT_X_kph  Table=MVMC_AggressLimitPCT_Y_pct  InternalRulePriority=Speed  RndMeth=Simplest  InputSameDT=on
  MVMC_SoftJerkPCT_pct : Lookup_n-D  NumberOfTableDimensions=1  BreakpointsForDimension1=AVMC_SoftJerkPCT_X_kph  Table=MVMC_SoftJerkPCT_Y_pct  InternalRulePriority=Speed  RndMeth=Simplest  InputSameDT=on
  MVMC_SoftLimitPCT_pct : Lookup_n-D  NumberOfTableDimensions=1  BreakpointsForDimension1=AVMC_SoftLimitPCT_X_kph  Table=MVMC_SoftLimitPCT_Y_pct  InternalRulePriority=Speed  RndMeth=Simplest  InputSameDT=on
  Relational Operator : RelationalOperator  Operator=>  OutDataTypeStr=boolean  RndMeth=Simplest
  Relational Operator1 : RelationalOperator  Operator=>  OutDataTypeStr=boolean  RndMeth=Simplest
  Response Gain : Stateflow chart  TreatAsAtomicUnit=on
  Saturation Dynamic{1..4} (4 alike) : simulink/Discontinuities/Saturation Dynamic  OutMin=[]  OutMax=[]  OutDataTypeStr=Inherit: Same as second input  OutDataType=fixdt(1, 16)  OutScaling=2^-10  DoSatur=off
  Switch : Switch  Criteria=u2 > Threshold  Threshold=KVMC_Veh2MeterSpdLoBdy_kph
  Switch{1..4} (4 alike) : Switch  Criteria=u2 > Threshold
  VVMC_JerkPCT_pct : Outport
  VVMC_LimitPCT_pct : Outport  Port=2
  wires:
  MVMC_SoftJerkPCT_pct/1 -> Saturation Dynamic4/2
  Constant35/1 -> Saturation Dynamic4/3
  Constant36/1 -> Saturation Dynamic4/1
  Switch2/1 -> Saturation Dynamic2/2
  Constant33/1 -> Saturation Dynamic2/3
  Constant34/1 -> Saturation Dynamic2/1
  MVMC_SoftLimitPCT_pct/1 -> Saturation Dynamic1/2
  Constant31/1 -> Saturation Dynamic1/3
  Constant32/1 -> Saturation Dynamic1/1
  Constant29/1 -> Saturation Dynamic3/3
  Constant30/1 -> Saturation Dynamic3/1
  Saturation Dynamic3/1 -> [VVMC_AggressLimitPCT_pct]  "VVMC_AggressLimitPCT_pct"
  MVMC_AggressJerkPCT_pct/1 -> Switch2/3
  MVMC_AggressLimitPCT_pct/1 -> Switch1/3
  [VVMC_MeterIndSpeedForCalcu_kph] -> Relational Operator1/2
  [VDSC_DISCTargetSpd_kph] -> Relational Operator1/1
  Relational Operator1/1 -> Switch4/2
  MVMC_AggressJerkPCT_pct1/1 -> Switch4/1
  Switch4/1 -> Switch2/1
  Switch3/1 -> Switch1/1
  MVMC_AggressLimitPCT_pct1/1 -> Switch3/1
  Relational Operator/1 -> Switch3/2
  [VDSC_DISCTargetSpd_kph] -> Relational Operator/1
  [VVMC_MeterIndSpeedForCalcu_kph] -> Relational Operator/2
  VDSC_DISCTargetSpd_kph/1 -> [VDSC_DISCTargetSpd_kph]
  MVMC_AggressLimitPCT4AT_pct/1 -> Switch3/3
  [VDSC_AutoTurnMode_flg] -> Switch1/2
  MVMC_AggressJerkPCT4AT_pct/1 -> Switch4/3
  [VDSC_AutoTurnMode_flg] -> Switch2/2
  VDSC_AutoTurnMode_flg/1 -> [VDSC_AutoTurnMode_flg]
  Constant5/1 -> Response Gain/14(KVMC_MSAResponseAGSV_flg)
  Constant4/1 -> Response Gain/13(TRUE)
  Constant3/1 -> Response Gain/12(ENUM_FEATARBITRSTA_MSA)
  Constant2/1 -> Response Gain/8(ENUM_FEATARBITRSTA_CC)
  Constant1/1 -> Divide5/1
  [VVMC_VehicleSpeed_kph] -> Divide5/2, Divide8/1, Switch/2
  Divide5/1 -> Add4/2
  Add4/1 -> Switch/1
  Constant28/1 -> Divide8/2
  Divide8/1 -> Switch/3
  Constant23/1 -> Add4/1
  Response Gain/1(VVMC_JerkPCT_pct) -> [VVMC_JerkPCT_pct]
  [VDSC_DISCTurn_flg] -> Response Gain/1(VDSC_DISCTurn_flg)
  Response Gain/2(VVMC_LimitPCT_pct) -> [VVMC_LimitPCT_pct]
  VDSC_DISCTurn_flg/1 -> [VDSC_DISCTurn_flg]
  VVMC_FeatArbitrSta_enum/1 -> [VVMC_FeatArbitrSta_enum]
  [VVMC_FeatArbitrSta_enum] -> Response Gain/2(VVMC_FeatArbitrSta_enum)
  [VVMC_SoftJerkPCT_pct] -> Response Gain/3(VVMC_SoftJerkPCT_pct)
  [VVMC_AggressJerkPCT_pct] -> Response Gain/4(VVMC_AggressJerkPCT_pct)
  [VVMC_SoftLimitPCT_pct] -> Response Gain/5(VVMC_SoftLimitPCT_pct)
  [VVMC_AggressLimitPCT_pct] -> Response Gain/6(VVMC_AggressLimitPCT_pct)
  [VVMC_JerkPCT_pct] -> VVMC_JerkPCT_pct/1
  [VVMC_LimitPCT_pct] -> VVMC_LimitPCT_pct/1
  Constant13/1 -> Response Gain/7(ENUM_FEATARBITRSTA_DISC)
  Constant15/1 -> Response Gain/9(ZERO_FLOAT)
  Constant16/1 -> Response Gain/10(ENUM_DISCTURN_ACTIVE)
  Constant18/1 -> Response Gain/11(ENUM_FEATARBITRSTA_ACCDISC)
  VVMC_MeterIndSpeedForCalcu_kph/1 -> [VVMC_MeterIndSpeedForCalcu_kph]
  [VVMC_MeterIndSpeedForCalcu_kph] -> MVMC_AggressJerkPCT_pct1/1, MVMC_AggressJerkPCT_pct/1, MVMC_AggressJerkPCT4AT_pct/1, MVMC_SoftJerkPCT_pct/1
  Saturation Dynamic4/1 -> [VVMC_SoftJerkPCT_pct]  "VVMC_SoftJerkPCT_pct"
  Saturation Dynamic2/1 -> [VVMC_AggressJerkPCT_pct]  "VVMC_AggressJerkPCT_pct"
  Saturation Dynamic1/1 -> [VVMC_SoftLimitPCT_pct]  "VVMC_SoftLimitPCT_pct"
  Switch1/1 -> Saturation Dynamic3/2
  VVMC_FeatReqSpd_kph/1 -> [VVMC_FeatReqSpd_kph]
  [VVMC_FeatReqSpd_kph] -> Add/2
  Add/1 -> Abs/1
  Abs/1 -> MVMC_AggressLimitPCT_pct/1, MVMC_SoftLimitPCT_pct/1, MVMC_AggressLimitPCT_pct1/1, MVMC_AggressLimitPCT4AT_pct/1
  VVMC_VehicleSpeed_kph/1 -> [VVMC_VehicleSpeed_kph]
  Switch/1 -> Add/1

== system vmc/VMC/VMC/ACC_Function/ACC Torque Source Determination/Triggered Subsystem2 ==
  In1 : Inport
  Trigger : TriggerPort  VariantControl=(inherit)
  Out1 : Outport
  wires:
  In1/1 -> Out1/1

== system vmc/VMC/VMC/ACC_Function/ACC Wheel Torque Calculation/Triggered Subsystem ==
  In1 : Inport
  Trigger : TriggerPort  VariantControl=(inherit)
  Out1 : Outport
  wires:
  In1/1 -> Out1/1

== system vmc/VMC/VMC/ACC_Function/ACC Wheel Torque Calculation/Triggered Subsystem1 ==
  In1 : Inport
  In2 : Inport  Port=2
  Trigger : TriggerPort  VariantControl=(inherit)
  Out1 : Outport
  Out2 : Outport  Port=2
  wires:
  In2/1 -> Out2/1
  In1/1 -> Out1/1

== system vmc/VMC/VMC/ACC_Function/ACC Wheel Torque Calculation/Triggered Subsystem2 ==
  In1 : Inport
  Trigger : TriggerPort  VariantControl=(inherit)
  Out1 : Outport
  wires:
  In1/1 -> Out1/1

== system vmc/VMC/VMC/ACC_Function/ACC Wheel Torque Calculation/Triggered Subsystem4 ==
  In1 : Inport
  Trigger : TriggerPort  VariantControl=(inherit)
  Out1 : Outport
  wires:
  In1/1 -> Out1/1

== system vmc/VMC/VMC/ACC_Function/ACC Wheel Torque Calculation/Triggered Subsystem5 ==
  In1 : Inport
  In2 : Inport  Port=2
  Trigger : TriggerPort  VariantControl=(inherit)
  Out1 : Outport
  Out2 : Outport  Port=2
  wires:
  In1/1 -> Out1/1
  In2/1 -> Out2/1

== system vmc/VMC/VMC/ACC_Function/ACC Wheel Torque Calculation/Triggered Subsystem6 ==
  In1 : Inport
  In2 : Inport  Port=2
  Trigger : TriggerPort  VariantControl=(inherit)
  Out1 : Outport
  Out2 : Outport  Port=2
  wires:
  In1/1 -> Out1/1
  In2/1 -> Out2/1

== system vmc/VMC/VMC/APS function/Signal Rounting/Signal Determination VINP_APSDecReqAtest_flg ==
  SignalInput1 : Inport
  SignalInput2 : Inport  Port=2
  VINP_SCPSystemMode_enum : Inport  Port=3
  VVMC_APSActive_flg : Inport  Port=4
  VVMC_ADASActive_flg : Inport  Port=5
  VVMC_CAASActive_flg : Inport  Port=6
  AND : Logic  Inputs=3  AllPortsSameDT=off  OutDataTypeStr=boolean
  Constant1 : Constant  Value=ENUM_SYSMODE_PRODUCT
  Constant3 : Constant  Value=KVMC_APSDevelopeSW_flg
  Equal : RelationalOperator  Operator===  OutDataTypeStr=boolean  RndMeth=Simplest
  OR : Logic  Operator=OR  Inputs=3  AllPortsSameDT=off  OutDataTypeStr=boolean
  Switch : Switch  Criteria=u2 > Threshold
  SignalOutp : Outport
  wires:
  VVMC_CAASActive_flg/1 -> OR/3
  Constant1/1 -> Equal/2
  Constant3/1 -> AND/2
  SignalInput2/1 -> Switch/3
  SignalInput1/1 -> Switch/1
  Switch/1 -> SignalOutp/1
  VINP_SCPSystemMode_enum/1 -> Equal/1
  Equal/1 -> AND/1
  VVMC_APSActive_flg/1 -> AND/3
  OR/1 -> Switch/2
  AND/1 -> OR/1
  VVMC_ADASActive_flg/1 -> OR/2

== system vmc/VMC/VMC/APS function/Signal Rounting/Signal Determination VINP_APSDecReqtest_mps2 ==
  SignalInput1 : Inport
  SignalInput2 : Inport  Port=2
  VINP_SCPSystemMode_enum : Inport  Port=3
  VVMC_APSActive_flg : Inport  Port=4
  VVMC_ADASActive_flg : Inport  Port=5
  VVMC_CAASActive_flg : Inport  Port=6
  AND : Logic  Inputs=3  AllPortsSameDT=off  OutDataTypeStr=boolean
  Constant1 : Constant  Value=ENUM_SYSMODE_PRODUCT
  Constant3 : Constant  Value=KVMC_APSDevelopeSW_flg
  Equal : RelationalOperator  Operator===  OutDataTypeStr=boolean  RndMeth=Simplest
  OR : Logic  Operator=OR  Inputs=3  AllPortsSameDT=off  OutDataTypeStr=boolean
  Switch : Switch  Criteria=u2 > Threshold
  SignalOutp : Outport
  wires:
  VVMC_CAASActive_flg/1 -> OR/3
  VVMC_ADASActive_flg/1 -> OR/2
  AND/1 -> OR/1
  OR/1 -> Switch/2
  VVMC_APSActive_flg/1 -> AND/3
  Equal/1 -> AND/1
  VINP_SCPSystemMode_enum/1 -> Equal/1
  Switch/1 -> SignalOutp/1
  SignalInput1/1 -> Switch/1
  SignalInput2/1 -> Switch/3
  Constant3/1 -> AND/2
  Constant1/1 -> Equal/2

== system vmc/VMC/VMC/APS function/Signal Rounting/Signal Determination VINP_APSReqtest_enum ==
  SignalInput1 : Inport
  SignalInput2 : Inport  Port=2
  VINP_SCPSystemMode_enum : Inport  Port=3
  VVMC_APSActive_flg : Inport  Port=4
  VVMC_ADASActive_flg : Inport  Port=5
  VVMC_CAASActive_flg : Inport  Port=6
  AND : Logic  Inputs=3  AllPortsSameDT=off  OutDataTypeStr=boolean
  Constant1 : Constant  Value=ENUM_SYSMODE_PRODUCT
  Constant3 : Constant  Value=KVMC_APSDevelopeSW_flg
  Equal : RelationalOperator  Operator===  OutDataTypeStr=boolean  RndMeth=Simplest
  OR : Logic  Operator=OR  Inputs=3  AllPortsSameDT=off  OutDataTypeStr=boolean
  Switch : Switch  Criteria=u2 > Threshold
  SignalOutp : Outport
  wires:
  VVMC_CAASActive_flg/1 -> OR/3
  Constant1/1 -> Equal/2
  Constant3/1 -> AND/2
  SignalInput2/1 -> Switch/3
  SignalInput1/1 -> Switch/1
  Switch/1 -> SignalOutp/1
  VINP_SCPSystemMode_enum/1 -> Equal/1
  Equal/1 -> AND/1
  VVMC_APSActive_flg/1 -> AND/3
  OR/1 -> Switch/2
  AND/1 -> OR/1
  VVMC_ADASActive_flg/1 -> OR/2

== system vmc/VMC/VMC/APS function/Signal Rounting/Signal Determination VINP_APSStaSystemtest_enum ==
  SignalInput1 : Inport
  SignalInput2 : Inport  Port=2
  VINP_SCPSystemMode_enum : Inport  Port=3
  VVMC_APSActive_flg : Inport  Port=4
  VVMC_ADASActive_flg : Inport  Port=5
  VTQD_GearActualPosn_enum : Inport  Port=6
  VVMC_CAASActive_flg : Inport  Port=7
  AND : Logic  Inputs=3  AllPortsSameDT=off  OutDataTypeStr=boolean
  AND1 : Logic  AllPortsSameDT=off  OutDataTypeStr=boolean
  Constant1 : Constant  Value=ENUM_SYSMODE_PRODUCT
  Constant2 : Constant  Value=ENUM_GEARACTUALPOSN_P
  Constant3 : Constant  Value=KVMC_APSDevelopeSW_flg
  Constant4 : Constant  Value=ENUM_APSSYSTEMSTA_ENABLE
  Constant5 : Constant  Value=KVMC_APSStaSystemOvrd_flg
  Equal : RelationalOperator  Operator===  OutDataTypeStr=boolean  RndMeth=Simplest
  Equal1 : RelationalOperator  Operator===  OutDataTypeStr=boolean  RndMeth=Simplest
  Equal2 : RelationalOperator  Operator===  OutDataTypeStr=boolean  RndMeth=Simplest
  OR : Logic  Operator=OR  Inputs=5  AllPortsSameDT=off  OutDataTypeStr=boolean
  Switch : Switch  Criteria=u2 > Threshold
  SignalOutp : Outport
  wires:
  VVMC_CAASActive_flg/1 -> OR/5
  Constant5/1 -> OR/4
  AND1/1 -> OR/3
  Constant4/1 -> Equal2/2
  [VINP_APSStaSystem_enum] -> Equal2/1
  Equal2/1 -> AND1/2
  Equal1/1 -> AND1/1
  Constant2/1 -> Equal1/2
  VTQD_GearActualPosn_enum/1 -> Equal1/1
  VVMC_ADASActive_flg/1 -> OR/2
  AND/1 -> OR/1
  OR/1 -> Switch/2
  VVMC_APSActive_flg/1 -> AND/3
  Equal/1 -> AND/1
  VINP_SCPSystemMode_enum/1 -> Equal/1
  Switch/1 -> SignalOutp/1
  SignalInput1/1 -> [VINP_APSStaSystem_enum], Switch/1
  SignalInput2/1 -> Switch/3
  Constant3/1 -> AND/2
  Constant1/1 -> Equal/2

== system vmc/VMC/VMC/Long Acceleration Calculation/Estimate Slope1/DelayEnable ==
  trigger : Inport
  T_delay : Inport  Port=2
  Ts : Inport  Port=3
  Constant1 : Constant  Value=ZERO_FLOAT
  Constant2 : Constant  Value=ZERO_FLOAT
  Relational Operator1 : RelationalOperator  Operator=>  OutDataTypeStr=boolean  RndMeth=Nearest
  Subtract1 : Sum
  Switch : Switch  Criteria=u2 ~= 0
      settings: AttributesFormatString=<%<Criteria>>
  Switch1 : Switch  Criteria=u2 ~= 0
      settings: AttributesFormatString=<%<Criteria>>
  Unit Delay : UnitDelay  SampleTime=-1  HasFrameUpgradeWarning=on
      settings: AttributesFormatString=<intial = %<X0>>
  Unit Delay1 : UnitDelay  InitialCondition=FALSE  SampleTime=-1  HasFrameUpgradeWarning=on
      settings: AttributesFormatString=<intial = %<X0>>
  set : Outport
  wires:
  Unit Delay1/1 -> Switch1/2
  Constant2/1 -> Switch1/1
  Ts/1 -> Switch1/3
  Switch1/1 -> Subtract1/2
  Unit Delay/1 -> Subtract1/1
  Relational Operator1/1 -> Unit Delay1/1, set/1
  trigger/1 -> Switch/2
  T_delay/1 -> Relational Operator1/2
  Constant1/1 -> Switch/3
  Switch/1 -> Unit Delay/1, Relational Operator1/1
  Subtract1/1 -> Switch/1

== system vmc/VMC/VMC/Long Acceleration Calculation/Estimate Slope1/DelayEnable4 ==
  trigger : Inport
  T_delay : Inport  Port=2
  Ts : Inport  Port=3
  Constant1 : Constant  Value=ZERO_FLOAT
  Constant2 : Constant  Value=ZERO_FLOAT
  Relational Operator1 : RelationalOperator  Operator=>  OutDataTypeStr=boolean  RndMeth=Nearest
  Subtract1 : Sum
  Switch : Switch  Criteria=u2 ~= 0
      settings: AttributesFormatString=<%<Criteria>>
  Switch1 : Switch  Criteria=u2 ~= 0
      settings: AttributesFormatString=<%<Criteria>>
  Unit Delay : UnitDelay  SampleTime=-1  HasFrameUpgradeWarning=on
      settings: AttributesFormatString=<intial = %<X0>>
  Unit Delay1 : UnitDelay  InitialCondition=FALSE  SampleTime=-1  HasFrameUpgradeWarning=on
      settings: AttributesFormatString=<intial = %<X0>>
  set : Outport
  wires:
  Unit Delay1/1 -> Switch1/2
  Constant2/1 -> Switch1/1
  Ts/1 -> Switch1/3
  Switch1/1 -> Subtract1/2
  Unit Delay/1 -> Subtract1/1
  Relational Operator1/1 -> Unit Delay1/1, set/1
  trigger/1 -> Switch/2
  T_delay/1 -> Relational Operator1/2
  Constant1/1 -> Switch/3
  Switch/1 -> Unit Delay/1, Relational Operator1/1
  Subtract1/1 -> Switch/1

== system vmc/VMC/VMC/Long Acceleration Calculation/Estimate Slope1/FirstOrderFilter3 ==
  in : Inport
  Tc : Inport  Port=2
  Ts : Inport  Port=3
  Add : Sum
  Add2 : Sum  Inputs=+-
  Constant3 : Constant  OutDataTypeStr=single
  Constant4 : Constant  Value=0  OutDataTypeStr=single
  Constant5 : Constant  Value=0  OutDataTypeStr=single
  Constant6 : Constant  Value=eps  OutDataTypeStr=single
  Divide : Product  Inputs=*/
  MinMax{1..4} (4 alike) : MinMax  Function=max  Inputs=2
  Product : Product  RndMeth=Zero
  Product1 : Product  RndMeth=Zero
  Unit Delay : UnitDelay  SampleTime=-1  HasFrameUpgradeWarning=on
  out : Outport
  wires:
  Add/1 -> out/1, Unit Delay/1
  Divide/1 -> Product1/1, Add2/2
  Constant3/1 -> Add2/1
  Add2/1 -> Product/2
  Product/1 -> Add/1
  Unit Delay/1 -> Product/1
  in/1 -> Product1/2
  Product1/1 -> Add/2
  Tc/1 -> MinMax2/1
  Constant4/1 -> MinMax2/2
  Ts/1 -> MinMax3/1
  Constant5/1 -> MinMax3/2
  MinMax3/1 -> MinMax1/2
  MinMax2/1 -> Divide/1, MinMax1/1
  MinMax1/1 -> MinMax4/1
  Constant6/1 -> MinMax4/2
  MinMax4/1 -> Divide/2

== system vmc/VMC/VMC/Long Acceleration Calculation/Estimate Slope1/FirstOrderFilter4 ==
  in : Inport
  Tc : Inport  Port=2
  Ts : Inport  Port=3
  Add : Sum
  Add2 : Sum  Inputs=+-
  Constant3 : Constant  OutDataTypeStr=single
  Constant4 : Constant  Value=0  OutDataTypeStr=single
  Constant5 : Constant  Value=0  OutDataTypeStr=single
  Constant6 : Constant  Value=eps  OutDataTypeStr=single
  Divide : Product  Inputs=*/
  MinMax{1..4} (4 alike) : MinMax  Function=max  Inputs=2
  Product : Product  RndMeth=Zero
  Product1 : Product  RndMeth=Zero
  Unit Delay : UnitDelay  SampleTime=-1  HasFrameUpgradeWarning=on
  out : Outport
  wires:
  Add/1 -> out/1, Unit Delay/1
  Divide/1 -> Product1/1, Add2/2
  Constant3/1 -> Add2/1
  Add2/1 -> Product/2
  Product/1 -> Add/1
  Unit Delay/1 -> Product/1
  in/1 -> Product1/2
  Product1/1 -> Add/2
  Tc/1 -> MinMax2/1
  Constant4/1 -> MinMax2/2
  Ts/1 -> MinMax3/1
  Constant5/1 -> MinMax3/2
  MinMax3/1 -> MinMax1/2
  MinMax2/1 -> Divide/1, MinMax1/1
  MinMax1/1 -> MinMax4/1
  Constant6/1 -> MinMax4/2
  MinMax4/1 -> Divide/2

== system vmc/VMC/VMC/Long Acceleration Calculation/Estimate Slope1/FirstOrderFilter5 ==
  in : Inport
  Tc : Inport  Port=2
  Ts : Inport  Port=3
  Add : Sum
  Add2 : Sum  Inputs=+-
  Constant3 : Constant  OutDataTypeStr=single
  Constant4 : Constant  Value=0  OutDataTypeStr=single
  Constant5 : Constant  Value=0  OutDataTypeStr=single
  Constant6 : Constant  Value=eps  OutDataTypeStr=single
  Divide : Product  Inputs=*/
  MinMax{1..4} (4 alike) : MinMax  Function=max  Inputs=2
  Product : Product  RndMeth=Zero
  Product1 : Product  RndMeth=Zero
  Unit Delay : UnitDelay  SampleTime=-1  HasFrameUpgradeWarning=on
  out : Outport
  wires:
  Add/1 -> out/1, Unit Delay/1
  Divide/1 -> Product1/1, Add2/2
  Constant3/1 -> Add2/1
  Add2/1 -> Product/2
  Product/1 -> Add/1
  Unit Delay/1 -> Product/1
  in/1 -> Product1/2
  Product1/1 -> Add/2
  Tc/1 -> MinMax2/1
  Constant4/1 -> MinMax2/2
  Ts/1 -> MinMax3/1
  Constant5/1 -> MinMax3/2
  MinMax3/1 -> MinMax1/2
  MinMax2/1 -> Divide/1, MinMax1/1
  MinMax1/1 -> MinMax4/1
  Constant6/1 -> MinMax4/2
  MinMax4/1 -> Divide/2

== system vmc/VMC/VMC/Long Acceleration Calculation/Estimate Slope1/FirstOrderFilter6 ==
  in : Inport
  Tc : Inport  Port=2
  Ts : Inport  Port=3
  Add : Sum
  Add2 : Sum  Inputs=+-
  Constant3 : Constant  OutDataTypeStr=single
  Constant4 : Constant  Value=0  OutDataTypeStr=single
  Constant5 : Constant  Value=0  OutDataTypeStr=single
  Constant6 : Constant  Value=eps  OutDataTypeStr=single
  Divide : Product  Inputs=*/
  MinMax{1..4} (4 alike) : MinMax  Function=max  Inputs=2
  Product : Product  RndMeth=Zero
  Product1 : Product  RndMeth=Zero
  Unit Delay : UnitDelay  SampleTime=-1  HasFrameUpgradeWarning=on
  out : Outport
  wires:
  Add/1 -> out/1, Unit Delay/1
  Divide/1 -> Product1/1, Add2/2
  Constant3/1 -> Add2/1
  Add2/1 -> Product/2
  Product/1 -> Add/1
  Unit Delay/1 -> Product/1
  in/1 -> Product1/2
  Product1/1 -> Add/2
  Tc/1 -> MinMax2/1
  Constant4/1 -> MinMax2/2
  Ts/1 -> MinMax3/1
  Constant5/1 -> MinMax3/2
  MinMax3/1 -> MinMax1/2
  MinMax2/1 -> Divide/1, MinMax1/1
  MinMax1/1 -> MinMax4/1
  Constant6/1 -> MinMax4/2
  MinMax4/1 -> Divide/2

== system vmc/VMC/VMC/Long Acceleration Calculation/Estimate Slope1/FirstOrderFilter7 ==
  in : Inport
  Tc : Inport  Port=2
  Ts : Inport  Port=3
  Add : Sum
  Add2 : Sum  Inputs=+-
  Constant3 : Constant  OutDataTypeStr=single
  Constant4 : Constant  Value=0  OutDataTypeStr=single
  Constant5 : Constant  Value=0  OutDataTypeStr=single
  Constant6 : Constant  Value=eps  OutDataTypeStr=single
  Divide : Product  Inputs=*/
  MinMax{1..4} (4 alike) : MinMax  Function=max  Inputs=2
  Product : Product  RndMeth=Zero
  Product1 : Product  RndMeth=Zero
  Unit Delay : UnitDelay  SampleTime=-1  HasFrameUpgradeWarning=on
  out : Outport
  wires:
  MinMax4/1 -> Divide/2
  Constant6/1 -> MinMax4/2
  MinMax1/1 -> MinMax4/1
  MinMax2/1 -> MinMax1/1, Divide/1
  MinMax3/1 -> MinMax1/2
  Constant5/1 -> MinMax3/2
  Ts/1 -> MinMax3/1
  Constant4/1 -> MinMax2/2
  Tc/1 -> MinMax2/1
  Product1/1 -> Add/2
  in/1 -> Product1/2
  Unit Delay/1 -> Product/1
  Product/1 -> Add/1
  Add2/1 -> Product/2
  Constant3/1 -> Add2/1
  Divide/1 -> Add2/2, Product1/1
  Add/1 -> Unit Delay/1, out/1

== system vmc/VMC/VMC/Long Acceleration Calculation/Estimate Slope1/FirstOrderFilter8 ==
  in : Inport
  Tc : Inport  Port=2
  Ts : Inport  Port=3
  Add : Sum
  Add2 : Sum  Inputs=+-
  Constant3 : Constant  OutDataTypeStr=single
  Constant4 : Constant  Value=0  OutDataTypeStr=single
  Constant5 : Constant  Value=0  OutDataTypeStr=single
  Constant6 : Constant  Value=eps  OutDataTypeStr=single
  Divide : Product  Inputs=*/
  MinMax{1..4} (4 alike) : MinMax  Function=max  Inputs=2
  Product : Product  RndMeth=Zero
  Product1 : Product  RndMeth=Zero
  Unit Delay : UnitDelay  SampleTime=-1  HasFrameUpgradeWarning=on
  out : Outport
  wires:
  Add/1 -> out/1, Unit Delay/1
  Divide/1 -> Product1/1, Add2/2
  Constant3/1 -> Add2/1
  Add2/1 -> Product/2
  Product/1 -> Add/1
  Unit Delay/1 -> Product/1
  in/1 -> Product1/2
  Product1/1 -> Add/2
  Tc/1 -> MinMax2/1
  Constant4/1 -> MinMax2/2
  Ts/1 -> MinMax3/1
  Constant5/1 -> MinMax3/2
  MinMax3/1 -> MinMax1/2
  MinMax2/1 -> Divide/1, MinMax1/1
  MinMax1/1 -> MinMax4/1
  Constant6/1 -> MinMax4/2
  MinMax4/1 -> Divide/2

== system vmc/VMC/VMC/Long Acceleration Calculation/Estimate Slope1/If Action Subsystem ==
  In1 : Inport
  Action Port : ActionPort
  Out1 : Outport
  wires:
  In1/1 -> Out1/1

== system vmc/VMC/VMC/Long Acceleration Calculation/Estimate Slope1/If Action Subsystem1 ==
  In1 : Inport
  Action Port : ActionPort
  Out1 : Outport
  wires:
  In1/1 -> Out1/1

== system vmc/VMC/VMC/Long Acceleration Calculation/Estimate Slope1/If Action Subsystem2 ==
  In1 : Inport
  Action Port : ActionPort
  Out1 : Outport
  wires:
  In1/1 -> Out1/1

== system vmc/VMC/VMC/Long Acceleration Calculation/Estimate Slope1/If Action Subsystem3 ==
  In1 : Inport
  Action Port : ActionPort
  Out1 : Outport
  wires:
  In1/1 -> Out1/1

== system vmc/VMC/VMC/Long Acceleration Calculation/Estimate Slope1/SR_Latch ==
  set : Inport
  reset : Inport  Port=2
  Data Type Conversion : DataTypeConversion  OutDataTypeStr=boolean
  Logical Operator : Logic  AllPortsSameDT=off  OutDataTypeStr=boolean
  Logical Operator1 : Logic  Operator=NOT  AllPortsSameDT=off  OutDataTypeStr=boolean
  Switch1 : Switch  Criteria=u2 ~= 0  Threshold=0.5
      settings: AttributesFormatString=<Criteria=%<Criteria>>
  Switch2 : Switch  Criteria=u2 ~= 0  Threshold=0.5
      settings: AttributesFormatString=<Criteria=%<Criteria>>
  Unit Delay : UnitDelay  SampleTime=-1  HasFrameUpgradeWarning=on
  latched : Outport
  wires:
  Logical Operator1/1 -> Switch2/1, Logical Operator/2
  Logical Operator/1 -> Switch1/2
  Switch2/1 -> Switch1/3
  Unit Delay/1 -> Switch2/3
  reset/1 -> Logical Operator1/1, Switch2/2
  set/1 -> Logical Operator/1, Switch1/1
  Switch1/1 -> Data Type Conversion/1
  Data Type Conversion/1 -> latched/1, Unit Delay/1
